simulink model "controller_testing_model"  (R2015a)
settings: Solver=ode3  StartTime=0.0  StopTime=20  RelTol=1e-3
values from neighbouring files (symbols this model uses):
  A = [3.98792656502 1 0 0 0 0 -5.81855146071 0 1 0 0 0 ... (36 elements, 6x6)]    [controller_params.mat]    (also in model_params.mat)
  B = [1 0 0 0 0 0]    [controller_params.mat]    (also in model_params.mat)
  C = [-0.000624151634985 0.000754210232314 -7.15793729404e-05 0 0 0]    [controller_params.mat]    (also in model_params.mat)
  M = [3543.77501475 3419.31647418 3291.64386704 3161.08265286 3028.02589994 2892.93065581]    [controller_params.mat]
  Nbar = 0.0315325549195    [controller_params.mat]    (also in controller_script.m = Nu + Kx*Nx; controller_script_lab_5.m = Nu + Kx*Nx)
  x_init = [0 0 0 0 0 0]    [controller_params.mat]    (also in controller_script.m = zeros(n_states, 1); controller_script_lab_5.m = zeros(n_states, 1))
undefined symbols (not defined in the file or in its folder): K, Ke, Kp, MIO, National_Instruments, PCI
libraries: sldrtlib x3
settings Model: SimulationMode=external  ExtModeTrigDuration=30001  Creator=Alunos  LastModifiedBy=Alunos
settings HardwareCC: ProdIntDivRoundTo=Zero  ProdEndianess=LittleEndian  ProdHWDeviceType=Intel->x86/Pentium  TargetIntDivRoundTo=Zero  TargetEndianess=LittleEndian  TargetHWDeviceType=Intel->x86/Pentium
settings RTWCC: SystemTargetFile=rtwin.tlc  TemplateMakefile=rtwin.tmf  Description=Simulink Desktop Real-Time  RTWCompilerOptimization=on
settings CodeAppCC: MaxIdLength=95
settings RTWinTargetCC: TargetPreCompLibLocation=C:\Program Files\MATLAB\R2015a\toolbox\sldrt\lib\win32

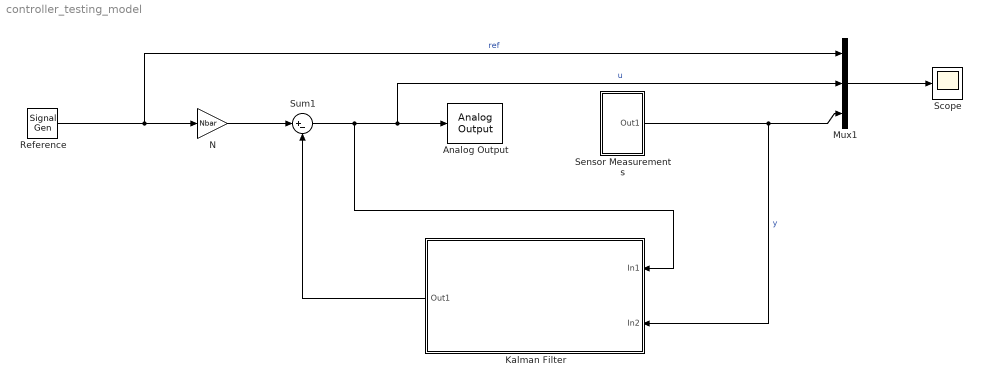
== system controller_testing_model ==
  Analog Output : sldrtlib/Analog Output  SampleTime=0.001  MaxMissedTicks=10  ShowMissedTicks=off  YieldWhenWaiting=off  DrvName=National_Instruments/PCI-MIO-16E-4  DrvAddress=4294967295  DrvOptions=[0 0 0 0 0 0]  Channels=1  RangeMode=1  VoltRange=1  InitialValue=0  FinalValue=0
      settings: AttributesFormatString=National Instruments\nPCI-MIO-16E-4 [auto]
  Kalman Filter : Subsystem
  Mux1 : Mux  Inputs=3
  N : Gain  Gain=Nbar
  Reference : SignalGenerator  WaveForm=square  Amplitude=30  Frequency=0.2
  Scope : Scope
      settings: ShowLegends=on
  Sensor Measurements : Subsystem
  Sum1 : Sum  Inputs=|+-
  wires:
  Sum1/1 -> Kalman Filter/1(In1), Analog Output/1, Mux1/2  "u"
  N/1 -> Sum1/1
  Sensor Measurements/1(Out1) -> Kalman Filter/2(In2), Mux1/3  "y"
  Kalman Filter/1(Out1) -> Sum1/2
  Reference/1 -> Mux1/1, N/1  "ref"
  Mux1/1 -> Scope/1

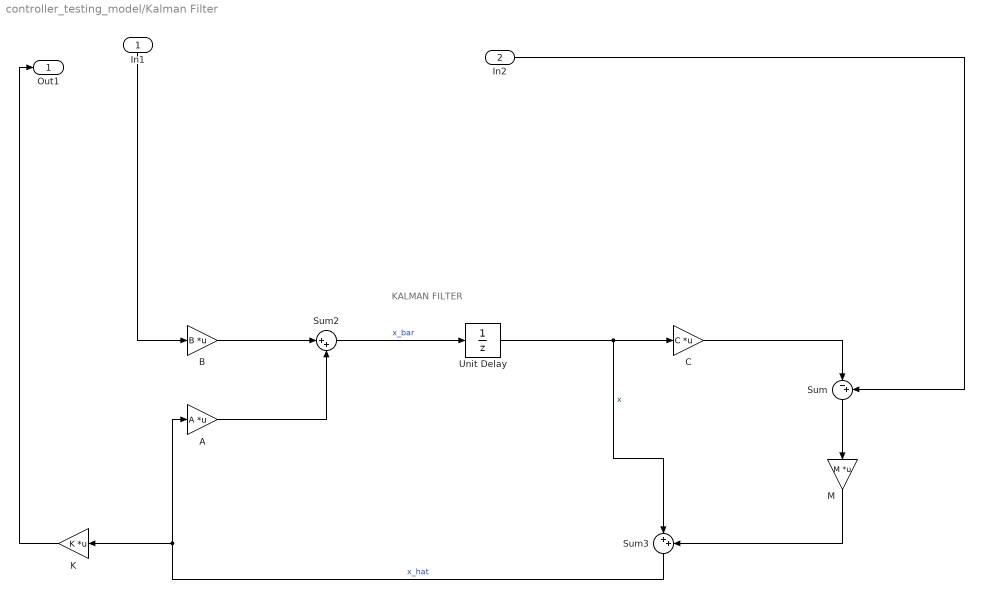
== system controller_testing_model/Kalman Filter ==
  note: KALMAN FILTER
  In1 : Inport
  In2 : Inport  Port=2
  A : Gain  Gain=A  Multiplication=Matrix(K*u)
  B : Gain  Gain=B  Multiplication=Matrix(K*u)
  C : Gain  Gain=C  Multiplication=Matrix(K*u)
  K : Gain  Gain=K  Multiplication=Matrix(K*u)
  M : Gain  Gain=M  Multiplication=Matrix(K*u)
  Sum : Sum  Inputs=|-+
  Sum2 : Sum  Inputs=|++
  Sum3 : Sum  Inputs=|++
  Unit Delay : UnitDelay  InitialCondition=x_init  SampleTime=0.001
  Out1 : Outport
  wires:
  M/1 -> Sum3/2
  Sum2/1 -> Unit Delay/1  "x_bar"
  A/1 -> Sum2/2
  B/1 -> Sum2/1
  Sum3/1 -> A/1, K/1  "x_hat"
  Sum/1 -> M/1
  In2/1 -> Sum/2
  C/1 -> Sum/1
  Unit Delay/1 -> C/1, Sum3/1  "x"
  K/1 -> Out1/1
  In1/1 -> B/1

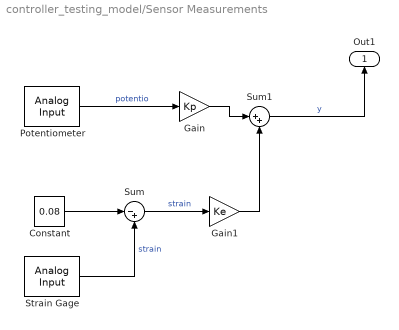
== system controller_testing_model/Sensor Measurements ==
  Constant : Constant  Value=0.08
  Gain : Gain  Gain=Kp
  Gain1 : Gain  Gain=Ke
  Potentiometer : sldrtlib/Analog Input  SampleTime=0.001  MaxMissedTicks=10  ShowMissedTicks=off  YieldWhenWaiting=off  DrvName=National_Instruments/PCI-MIO-16E-4  DrvAddress=4294967295  DrvOptions=[0 0 0 0 0 0]  Channels=1  RangeMode=1  VoltRange=1  DataType=1
      settings: AttributesFormatString=National Instruments\nPCI-MIO-16E-4 [auto]
  Strain Gage : sldrtlib/Analog Input  SampleTime=0.001  MaxMissedTicks=10  ShowMissedTicks=off  YieldWhenWaiting=off  DrvName=National_Instruments/PCI-MIO-16E-4  DrvAddress=4294967295  DrvOptions=[0 0 0 0 0 0]  Channels=2  RangeMode=1  VoltRange=1  DataType=1
      settings: AttributesFormatString=National Instruments\nPCI-MIO-16E-4 [auto]
  Sum : Sum  Inputs=|-+
  Sum1 : Sum  Inputs=|++
  Out1 : Outport
  wires:
  Potentiometer/1 -> Gain/1  "potentio"
  Constant/1 -> Sum/1
  Strain Gage/1 -> Sum/2  "strain"
  Sum/1 -> Gain1/1  "strain"
  Sum1/1 -> Out1/1  "y"
  Gain/1 -> Sum1/1
  Gain1/1 -> Sum1/2
